simulink model "filtersamy"  (R2023b)
settings: Solver=VariableStepAuto  StartTime=0.0  StopTime=10.0  RelTol=1e-3
values from neighbouring files (symbols this model uses):
  ts = 1/fs    (= 4e-05)    [FIR.m]    (also in FIRfiltSam.m)
settings Model: Creator=lekhanreddy  LastModifiedBy=91798

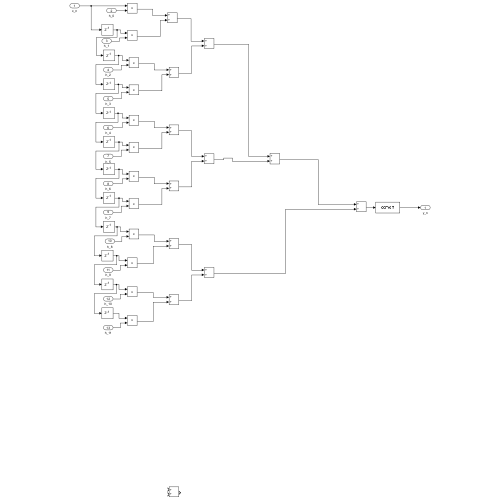
[thumbnail: Simulink's stored preview of the top-level diagram]
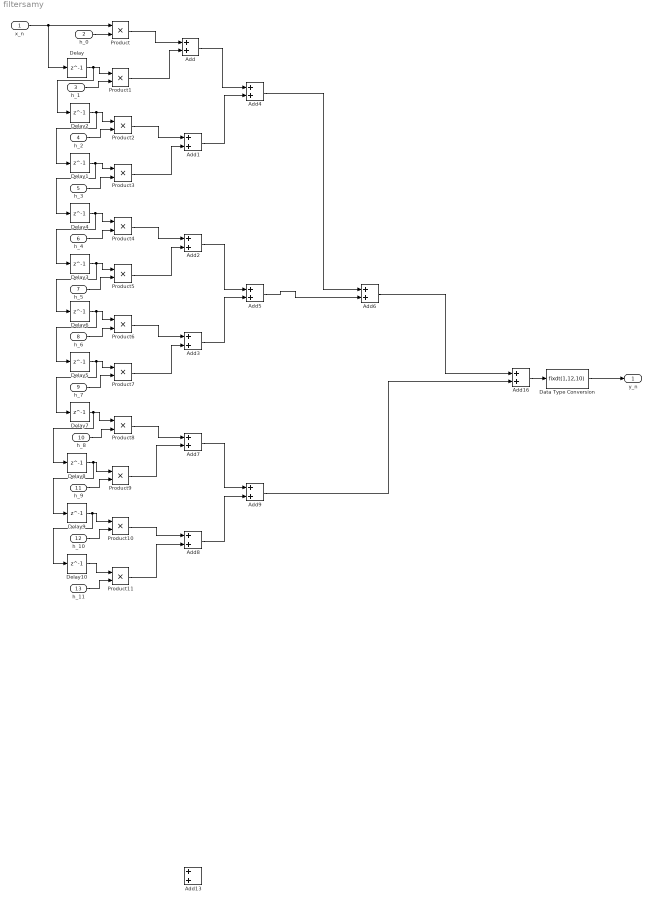
== system filtersamy ==
  x_n : Inport  OutDataTypeStr=fixdt(1,8,6)  SampleTime=ts
  h_0 : Inport  Port=2  OutDataTypeStr=fixdt(1,8,6)
  h_1 : Inport  Port=3  OutDataTypeStr=fixdt(1,8,6)
  h_2 : Inport  Port=4  OutDataTypeStr=fixdt(1,8,6)
  h_3 : Inport  Port=5  OutDataTypeStr=fixdt(1,8,6)
  h_4 : Inport  Port=6  OutDataTypeStr=fixdt(1,8,6)
  h_5 : Inport  Port=7  OutDataTypeStr=fixdt(1,8,6)
  h_6 : Inport  Port=8  OutDataTypeStr=fixdt(1,8,6)
  h_7 : Inport  Port=9  OutDataTypeStr=fixdt(1,8,6)
  h_8 : Inport  Port=10  OutDataTypeStr=fixdt(1,8,6)
  h_9 : Inport  Port=11  OutDataTypeStr=fixdt(1,8,6)
  h_10 : Inport  Port=12  OutDataTypeStr=fixdt(1,8,6)  SampleTime=ts
  h_11 : Inport  Port=13  OutDataTypeStr=fixdt(1,8,6)  SampleTime=ts
  Add{,1..9,13,16} (12 alike) : Sum
  Data Type Conversion : DataTypeConversion  OutDataTypeStr=fixdt(1,12,10)  SaturateOnIntegerOverflow=off  RndMeth=Floor
  Delay{,1..10} (11 alike) : Delay  DelayLength=1  InitialCondition=0
  Product{,1..11} (12 alike) : Product
  y_n : Outport  VectorParamsAs1DForOutWhenUnconnected=off
  wires:
  h_0/1 -> Product/2
  Product5/1 -> Add2/2
  h_3/1 -> Product3/2
  Product/1 -> Add/1
  Delay5/1 -> Delay7/1, Product7/1
  Product3/1 -> Add1/2
  h_5/1 -> Product5/2
  h_1/1 -> Product1/2
  Delay1/1 -> Delay4/1, Product3/1
  Product4/1 -> Add2/1
  Delay3/1 -> Delay6/1, Product5/1
  h_7/1 -> Product7/2
  Delay6/1 -> Delay5/1, Product6/1
  Add5/1 -> Add6/2
  Product2/1 -> Add1/1
  Product7/1 -> Add3/2
  Product6/1 -> Add3/1
  Delay2/1 -> Delay1/1, Product2/1
  h_6/1 -> Product6/2
  h_2/1 -> Product2/2
  Delay4/1 -> Delay3/1, Product4/1
  Product1/1 -> Add/2
  Add/1 -> Add4/1
  h_4/1 -> Product4/2
  Add1/1 -> Add4/2
  x_n/1 -> Delay/1, Product/1
  Add2/1 -> Add5/1
  Add3/1 -> Add5/2
  Add4/1 -> Add6/1
  Data Type Conversion/1 -> y_n/1
  Delay/1 -> Product1/1, Delay2/1
  h_8/1 -> Product8/2
  h_9/1 -> Product9/2
  Delay7/1 -> Delay8/1, Product8/1
  h_10/1 -> Product10/2
  Delay8/1 -> Delay9/1, Product9/1
  h_11/1 -> Product11/2
  Delay9/1 -> Delay10/1, Product10/1
  Delay10/1 -> Product11/1
  Product11/1 -> Add8/2
  Product9/1 -> Add7/2
  Add8/1 -> Add9/2
  Add7/1 -> Add9/1
  Product8/1 -> Add7/1
  Product10/1 -> Add8/1
  Add6/1 -> Add16/1
  Add16/1 -> Data Type Conversion/1
  Add9/1 -> Add16/2
